simulink model "test_discrete_minjerk_filter"  (R2025b)
settings: Solver=VariableStepAuto  StartTime=0.0  StopTime=7  RelTol=1e-3
model workspace (MAT data in the model file):
  Ts = Simulink.Parameter
  Ts.Value = 0.001
  Ts.Complexity = 'real'
  Ts.Dimensions = [1 1]
  Ts.Description = 'Sample time.'
  Ts.DataType = 'auto'
  Ts.DocUnits = 's'
libraries: simulink x2, arsenal x1, shareduavrstlib x1
settings Model: Creator=upattacini  LastModifiedBy=upattacini
settings DataIOCC: SaveOutput=off  DSMLogging=off  SaveTime=off  ReturnWorkspaceOutputs=off

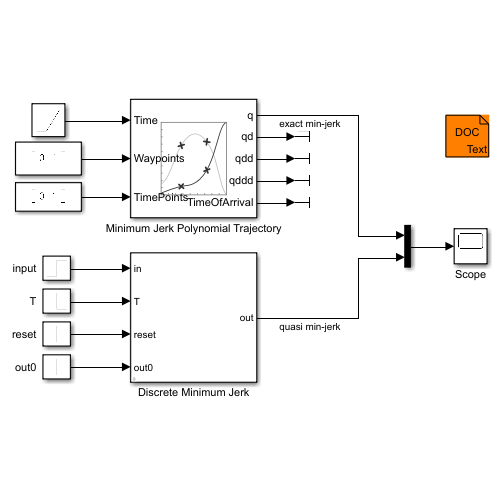
[thumbnail: Simulink's stored preview of the top-level diagram]
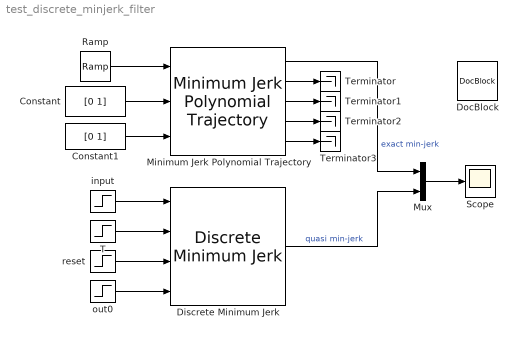
== system test_discrete_minjerk_filter ==
  Constant : Constant  Value=[0 1]  VectorParams1D=off
  Constant1 : Constant  Value=[0 1]  VectorParams1D=off
  Discrete Minimum Jerk : arsenal/Filters/Discrete Minimum Jerk  Ts=Ts
      settings: SourceProductName=MESH Arsenal
  DocBlock : simulink/Model-Wide Utilities/DocBlock  DocumentType=Text
      content=|
      | Discrete Minimum Jerk Filter
      | ============================
      |
      | - This discrete filter implements a quasi minimum jerk smoother.
      | - Remarkably, the filter's rise-time can be adjusted at runtime.
      | - The block is ready for code generation.
      |
      | The implementation is based on the paper https://ieeexplore.ieee.org/document/5650851.
  Minimum Jerk Polynomial Trajectory : shareduavrstlib/Minimum Jerk Polynomial Trajectory  ShowBCInputPort=off  ShowPolynomialCoefs=off  ShowStatusOutputPort=off  TimeAllocation=off  TimeWeight=100  MinSegmentTime=0.1  MaxSegmentTime=1  MaxIteration=1500  MaxTime=10  SimulateUsing=Code generation
      settings: LibrarySourceBlock=robotutilslib/Minimum Jerk Polynomial Trajectory
  Mux : Mux  Inputs=2
  Ramp : simulink/Sources/Ramp  slope=1  start=1  InitialOutput=0
  Scope : Scope
      settings: SampleTime=Ts  ActiveDisplayYMinimum=-0.24999998145200056  ActiveDisplayYMaximum=2.2499998330680056
  T : Step  Time=4  Before=1  After=0.5  SampleTime=0
  Terminator{,1..3} (4 alike) : Terminator
  input : Step  SampleTime=0
  out0 : Step  Time=4  After=2  SampleTime=0
  reset : Step  Time=4  SampleTime=0
  wires:
  Ramp/1 -> Minimum Jerk Polynomial Trajectory/1
  Constant/1 -> Minimum Jerk Polynomial Trajectory/2
  Constant1/1 -> Minimum Jerk Polynomial Trajectory/3
  Minimum Jerk Polynomial Trajectory/2 -> Terminator/1
  Minimum Jerk Polynomial Trajectory/3 -> Terminator1/1
  Minimum Jerk Polynomial Trajectory/4 -> Terminator2/1
  Minimum Jerk Polynomial Trajectory/5 -> Terminator3/1
  input/1 -> Discrete Minimum Jerk/1
  Minimum Jerk Polynomial Trajectory/1 -> Mux/1  "exact min-jerk"
  Discrete Minimum Jerk/1 -> Mux/2  "quasi min-jerk"
  Mux/1 -> Scope/1
  T/1 -> Discrete Minimum Jerk/2
  reset/1 -> Discrete Minimum Jerk/3
  out0/1 -> Discrete Minimum Jerk/4
